simulink model "Lab5_Sim"  (R2024a)
settings: Solver=FixedStepAuto  StartTime=0.0  StopTime=4717440  FixedStep=50  RelTol=1e-3
values from neighbouring files (symbols this model uses):
  G = 6.674e-11    [L_points.m]    (also in Lab3_Driver.m; Lab5.m; Lab8.m; LagrangePoints.m = 6.67408e-11)
  mE = 5.97219e24    (= 5.97219e+24)    [L_points.m]    (also in Lab5.m; Lab8.m; Presentation_Circular.m; Presentation_HaloOrbit.m)
  mM = 7.349e22    (= 7.349e+22)    [L_points.m]    (also in Lab5.m; Lab8.m; Presentation_Circular.m = plot3(OM(mid,1)/1000,OM(mid,2)/1000,OM(mid,3)/1000,Marker="o; Presentation_HaloOrbit.m)
  posE = [3.034529801433376E+03 -3.340359653273315E+03 -1.939037192252903E+03]*1000    [L_points.m]    (also in Lab5.m = [-xE 0 0]; Lab8.m = [-xE 0 0]; Presentation_Circular.m = [-xE 0 0]; Presentation_HaloOrbit.m = [-xE 0 0])
  posM = [-2.467089971416006E+05 3.118709928882247E+05 3.661070919281326E+04]*1000    [L_points.m]    (also in Lab5.m = [xM 0 0]; Lab8.m = [xM 0 0]; Presentation_Circular.m = [xM 0 0]; Presentation_HaloOrbit.m = [xM 0 0])
  posS = [-2.066118376482230E+05 4.155370802455372E+05 4.252060750636854E+04+3500]*1000    [L_points.m]    (also in Lab5.m = [xL2 yS 0]; Lab8.m = [xL2 0 zL2]; Presentation_Circular.m = [xL2 0 0]; Presentation_HaloOrbit.m = [xL2-400 0 2000])
  velE = [9.245683416082787E-03 6.608382937807280E-03 2.954691314042687E-03]*1000    [L_points.m]    (also in Lab5.m = [0 -vE 0]; Lab8.m = [0 -vE 0]; Presentation_Circular.m = [0 -vE 0]; Presentation_HaloOrbit.m = [0 -vE 0])
  velM = [-7.516793153236040E-01 -5.884845299522508E-01 -6.683923719039309E-03]*1000    [L_points.m]    (also in Lab5.m = [0 vM 0]; Lab8.m = [0 vM 0]; Presentation_Circular.m = [0 vM 0]; Presentation_HaloOrbit.m = [0 vM 0])
  velS = velM    [L_points.m]    (also in Lab5.m = [0 vSe -vSh]; Lab8.m = [0 vSe+vSh 0]; Presentation_Circular.m = [0 vSe 0]; Presentation_HaloOrbit.m = [-0.002 vSe+0.008 0])
settings Model: Creator=sgtjake2  LastModifiedBy=User

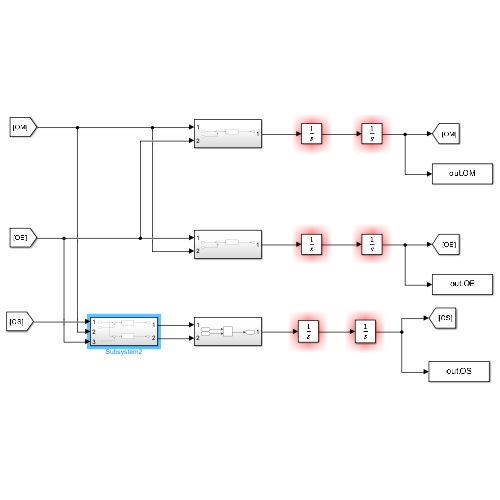
[thumbnail: Simulink's stored preview of the top-level diagram]
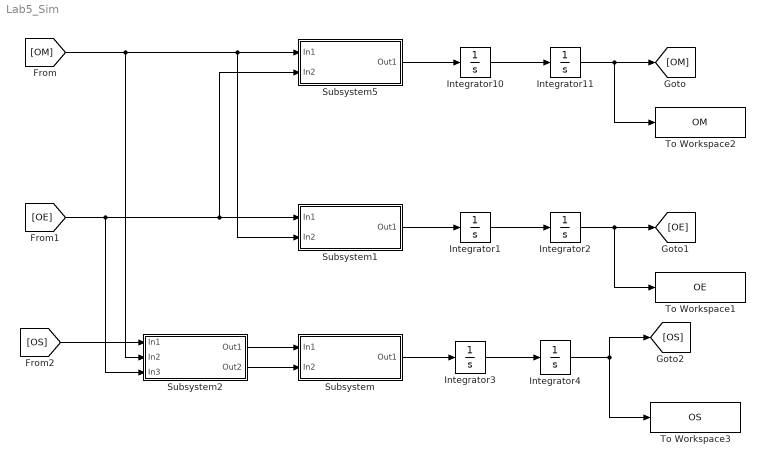
== system Lab5_Sim ==
  Integrator1 : Integrator  InitialCondition=velE
  Integrator10 : Integrator  InitialCondition=velM
  Integrator11 : Integrator  InitialCondition=posM
  Integrator2 : Integrator  InitialCondition=posE
  Integrator3 : Integrator  InitialCondition=velS
  Integrator4 : Integrator  InitialCondition=posS
  Subsystem : Subsystem
  Subsystem1 : Subsystem
  Subsystem2 : Subsystem
  Subsystem5 : Subsystem
  To Workspace1 : ToWorkspace  VariableName=OE  SaveFormat=Timeseries  SampleTime=-1
  To Workspace2 : ToWorkspace  VariableName=OM  SaveFormat=Timeseries  SampleTime=-1
  To Workspace3 : ToWorkspace  VariableName=OS  SaveFormat=Timeseries  SampleTime=-1
  wires:
  [OE] -> Subsystem2/3(In3), Subsystem1/1(In1), Subsystem5/2(In2)
  [OM] -> Subsystem1/2(In2), Subsystem5/1(In1), Subsystem2/2(In2)
  Integrator1/1 -> Integrator2/1
  Subsystem1/1(Out1) -> Integrator1/1
  Integrator11/1 -> To Workspace2/1, [OM]
  Subsystem5/1(Out1) -> Integrator10/1
  Integrator2/1 -> To Workspace1/1, [OE]
  Integrator10/1 -> Integrator11/1
  Integrator4/1 -> To Workspace3/1, [OS]
  Subsystem/1(Out1) -> Integrator3/1
  Subsystem2/2(Out2) -> Subsystem/2(In2)
  Subsystem2/1(Out1) -> Subsystem/1(In1)
  Integrator3/1 -> Integrator4/1
  [OS] -> Subsystem2/1(In1)

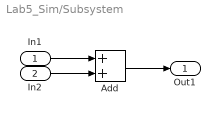
== system Lab5_Sim/Subsystem ==
  In1 : Inport
  In2 : Inport  Port=2
  Add : Sum
  Out1 : Outport
  wires:
  Add/1 -> Out1/1
  In1/1 -> Add/1
  In2/1 -> Add/2

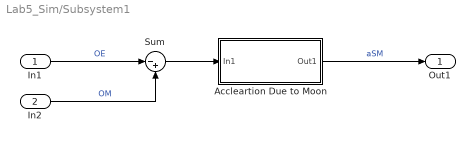
== system Lab5_Sim/Subsystem1 ==
  In1 : Inport
  In2 : Inport  Port=2
  Accleartion Due to Moon : Subsystem
  Sum : Sum  Inputs=|-+
  Out1 : Outport
  wires:
  Accleartion Due to Moon/1(Out1) -> Out1/1  "aSM"
  Sum/1 -> Accleartion Due to Moon/1(In1)
  In1/1 -> Sum/1  "OE"
  In2/1 -> Sum/2  "OM"

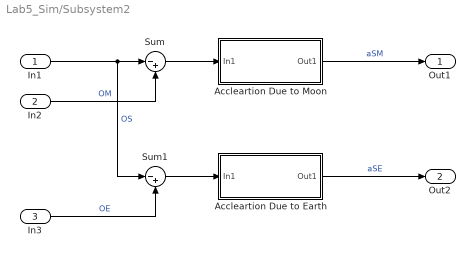
== system Lab5_Sim/Subsystem2 ==
  In1 : Inport
  In2 : Inport  Port=2
  In3 : Inport  Port=3
  Accleartion Due to Earth : Subsystem
  Accleartion Due to Moon : Subsystem
  Sum : Sum  Inputs=|-+
  Sum1 : Sum  Inputs=|-+
  Out1 : Outport
  Out2 : Outport  Port=2
  wires:
  Accleartion Due to Moon/1(Out1) -> Out1/1  "aSM"
  Sum/1 -> Accleartion Due to Moon/1(In1)
  In1/1 -> Sum1/1, Sum/1  "OS"
  In2/1 -> Sum/2  "OM"
  Sum1/1 -> Accleartion Due to Earth/1(In1)
  Accleartion Due to Earth/1(Out1) -> Out2/1  "aSE"
  In3/1 -> Sum1/2  "OE"

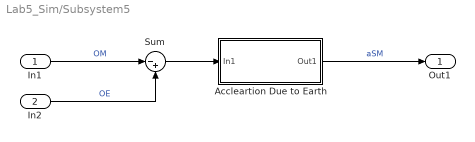
== system Lab5_Sim/Subsystem5 ==
  In1 : Inport
  In2 : Inport  Port=2
  Accleartion Due to Earth : Subsystem
  Sum : Sum  Inputs=|-+
  Out1 : Outport
  wires:
  Accleartion Due to Earth/1(Out1) -> Out1/1  "aSM"
  Sum/1 -> Accleartion Due to Earth/1(In1)
  In1/1 -> Sum/1  "OM"
  In2/1 -> Sum/2  "OE"

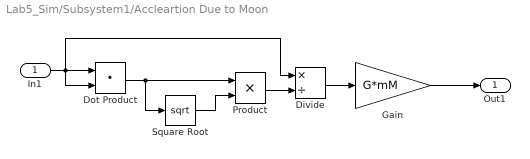
== system Lab5_Sim/Subsystem1/Accleartion Due to Moon ==
  In1 : Inport
  Divide : Product  Inputs=*/
  Dot Product : DotProduct  OutDataTypeStr=Inherit: Inherit via internal rule
  Gain : Gain  Gain=G*mM
  Product : Product
  Square Root : Sqrt
  Out1 : Outport
  wires:
  In1/1 -> Divide/1, Dot Product/2, Dot Product/1
  Dot Product/1 -> Square Root/1, Product/1
  Square Root/1 -> Product/2
  Product/1 -> Divide/2
  Gain/1 -> Out1/1
  Divide/1 -> Gain/1

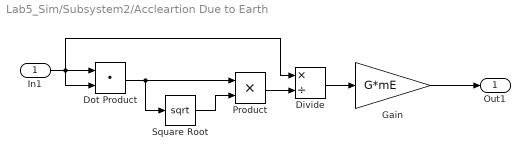
== system Lab5_Sim/Subsystem2/Accleartion Due to Earth ==
  In1 : Inport
  Divide : Product  Inputs=*/
  Dot Product : DotProduct  OutDataTypeStr=Inherit: Inherit via internal rule
  Gain : Gain  Gain=G*mE
  Product : Product
  Square Root : Sqrt
  Out1 : Outport
  wires:
  In1/1 -> Divide/1, Dot Product/2, Dot Product/1
  Dot Product/1 -> Square Root/1, Product/1
  Square Root/1 -> Product/2
  Product/1 -> Divide/2
  Gain/1 -> Out1/1
  Divide/1 -> Gain/1

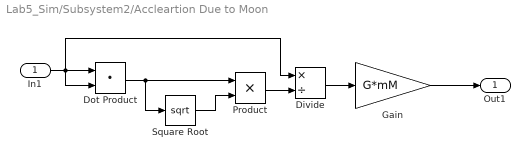
== system Lab5_Sim/Subsystem2/Accleartion Due to Moon ==
  In1 : Inport
  Divide : Product  Inputs=*/
  Dot Product : DotProduct  OutDataTypeStr=Inherit: Inherit via internal rule
  Gain : Gain  Gain=G*mM
  Product : Product
  Square Root : Sqrt
  Out1 : Outport
  wires:
  In1/1 -> Divide/1, Dot Product/2, Dot Product/1
  Dot Product/1 -> Square Root/1, Product/1
  Square Root/1 -> Product/2
  Product/1 -> Divide/2
  Gain/1 -> Out1/1
  Divide/1 -> Gain/1

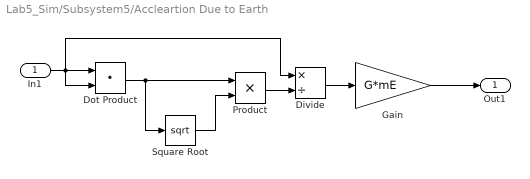
== system Lab5_Sim/Subsystem5/Accleartion Due to Earth ==
  In1 : Inport
  Divide : Product  Inputs=*/
  Dot Product : DotProduct  OutDataTypeStr=Inherit: Inherit via internal rule
  Gain : Gain  Gain=G*mE
  Product : Product
  Square Root : Sqrt
  Out1 : Outport
  wires:
  In1/1 -> Divide/1, Dot Product/2, Dot Product/1
  Dot Product/1 -> Square Root/1, Product/1
  Square Root/1 -> Product/2
  Product/1 -> Divide/2
  Gain/1 -> Out1/1
  Divide/1 -> Gain/1
